simulink model "antiwindup"  (R2023a)
settings: Solver=VariableStepAuto  StartTime=0.0  StopTime=10.0  RelTol=1e-3
values from neighbouring files (symbols this model uses):
  Kid = acker(DAamp, DBamp, [exp(- p * T), exp(-0.5 * p * T), exp(-0.7*p*T)])    [discretizar.m]
  Ld = acker(sysd.A', C', [exp(-1.2*p * T), exp(-1.2 * p * T)] )'    [discretizar.m]
  sysd = c2d(sys, T)    [discretizar.m]
  T = 1e-4    (= 0.0001)    [discretizar.m]
undefined symbols (not defined in the file or in its folder): C, ke, p
settings Model: Creator=erwinplanck  LastModifiedBy=erwinplanck

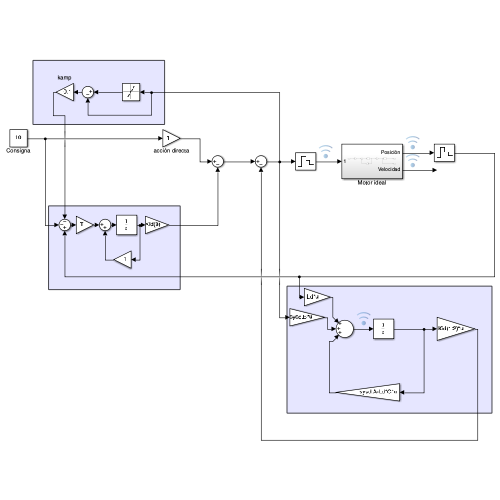
[thumbnail: Simulink's stored preview of the top-level diagram]
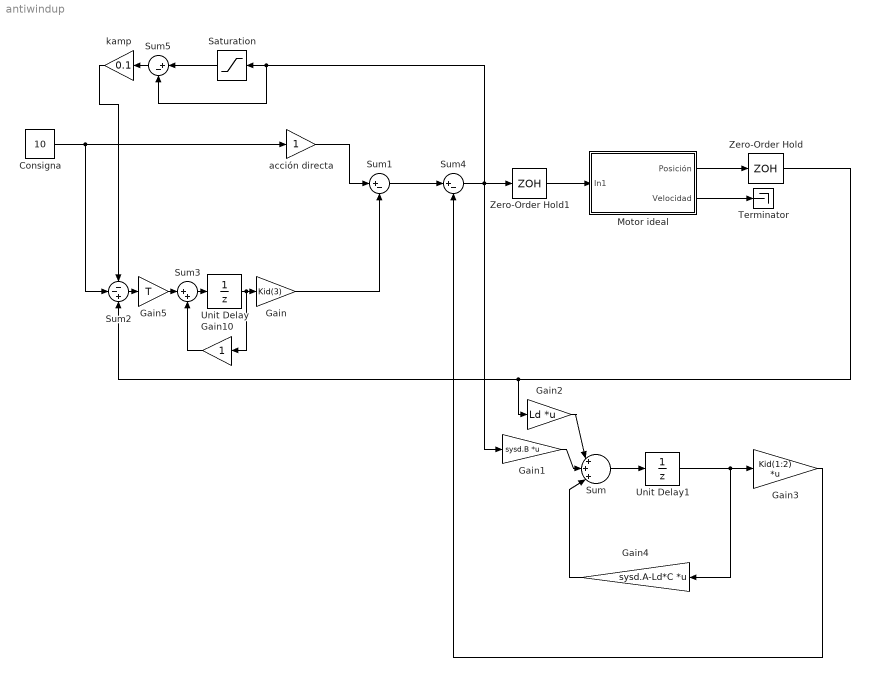
== system antiwindup ==
  Consigna : Constant  Value=10
  Gain : Gain  Gain=Kid(3)
  Gain1 : Gain  Gain=sysd.B  Multiplication=Matrix(K*u)
  Gain10 : Gain
  Gain2 : Gain  Gain=Ld  Multiplication=Matrix(K*u)
  Gain3 : Gain  Gain=Kid(1:2)  Multiplication=Matrix(K*u)
  Gain4 : Gain  Gain=sysd.A-Ld*C  Multiplication=Matrix(K*u)
  Gain5 : Gain  Gain=T
  Motor ideal : Subsystem
  Saturation : Saturate  UpperLimit=12  LowerLimit=-12
  Sum : Sum  Inputs=|+++|
  Sum1 : Sum  Inputs=|+-
  Sum2 : Sum  Inputs=--+
  Sum3 : Sum  Inputs=|++
  Sum4 : Sum  Inputs=|+-
  Sum5 : Sum  Inputs=|+-
  Terminator : Terminator
  Unit Delay : UnitDelay  SampleTime=T  HasFrameUpgradeWarning=on
  Unit Delay1 : UnitDelay  SampleTime=T  HasFrameUpgradeWarning=on
  Zero-Order Hold : ZeroOrderHold  SampleTime=T
  Zero-Order Hold1 : ZeroOrderHold  SampleTime=T
  acción directa : Gain
  kamp : Gain  Gain=0.1
  wires:
  Sum3/1 -> Unit Delay/1
  Gain4/1 -> Sum/3
  Sum1/1 -> Sum4/1
  Gain3/1 -> Sum4/2
  Motor ideal/2(Velocidad) -> Terminator/1
  Consigna/1 -> acción directa/1, Sum2/2
  Gain/1 -> Sum1/2
  acción directa/1 -> Sum1/1
  Motor ideal/1(Posición) -> Zero-Order Hold/1
  Gain1/1 -> Sum/2
  Gain10/1 -> Sum3/2
  Unit Delay1/1 -> Gain4/1, Gain3/1
  Sum2/1 -> Gain5/1
  Gain5/1 -> Sum3/1
  Gain2/1 -> Sum/1
  Sum/1 -> Unit Delay1/1
  Unit Delay/1 -> Gain10/1, Gain/1
  Sum4/1 -> Gain1/1, Sum5/2, Saturation/1, Zero-Order Hold1/1
  Zero-Order Hold1/1 -> Motor ideal/1(In1)
  Zero-Order Hold/1 -> Sum2/3, Gain2/1
  Saturation/1 -> Sum5/1
  Sum5/1 -> kamp/1
  kamp/1 -> Sum2/1

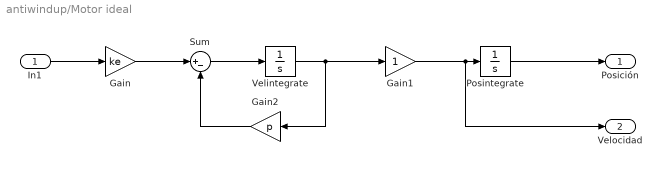
== system antiwindup/Motor ideal ==
  In1 : Inport
  Gain : Gain  Gain=ke
  Gain1 : Gain
  Gain2 : Gain  Gain=p
  Posintegrate : Integrator
  Sum : Sum  Inputs=|+-
  Velintegrate : Integrator  InitialCondition=4
  Posición : Outport
  Velocidad : Outport  Port=2
  wires:
  Sum/1 -> Velintegrate/1
  Gain2/1 -> Sum/2
  Gain1/1 -> Velocidad/1, Posintegrate/1
  Posintegrate/1 -> Posición/1
  In1/1 -> Gain/1
  Velintegrate/1 -> Gain2/1, Gain1/1
  Gain/1 -> Sum/1
